simulink model "PI"  (R2020b)
settings: Solver=VariableStepAuto  StartTime=0.0  StopTime=300.0  RelTol=1e-3
values from neighbouring files (symbols this model uses):
  Kp = (0.9*T0)/(K0*(tau + 0.5*T)) - (0.5*Ki)/K0    (= 0.670050069403)    [Parametri_PI.m]    (also in Parametri_PID.m = 0.886775962404)
  T = 0.01    [Parametri_PI.m]    (also in Parametri_PID.m)
  Ti = (Kp*T)/Ki    (= 2.4575)    [Parametri_PI.m]    (also in Parametri_PID.m = 1.46356729475)
libraries: simulink x1
settings Model: Creator=user  LastModifiedBy=user

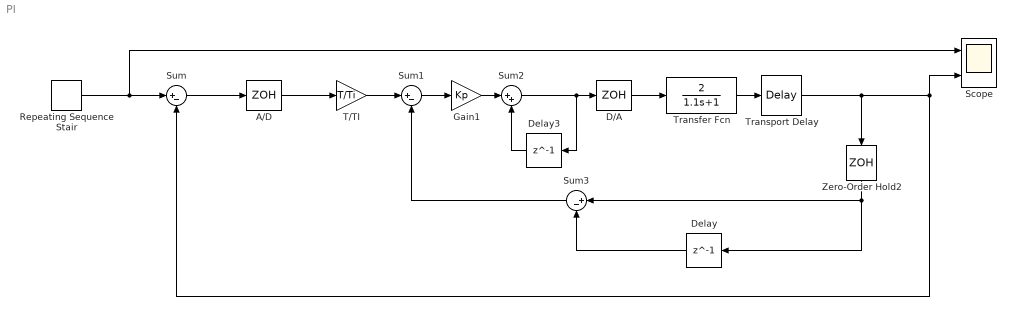
== system PI ==
  A/D : ZeroOrderHold  SampleTime=0.01
  D/A : ZeroOrderHold  SampleTime=0.01
  Delay : Delay  DelayLength=1
  Delay3 : Delay  DelayLength=1
  Gain1 : Gain  Gain=Kp
  Repeating Sequence Stair : simulink/Sources/Repeating Sequence Stair  OutValues=[3 1 -5 2 1].'  tsamp=50  OutMin=[]  OutMax=[]  OutDataTypeStr=double  OutputDataTypeScalingMode=double  OutDataType=fixdt(0,8)  ConRadixGroup=Best Precision: Vector-wise  OutScaling=2^-12
  Scope : Scope  NumInputPorts=2
  Sum : Sum  Inputs=|+-
  Sum1 : Sum  Inputs=|+-
  Sum2 : Sum  Inputs=|++
  Sum3 : Sum  Inputs=|+-
  T/TI : Gain  Gain=T/Ti
  Transfer Fcn : TransferFcn  Numerator=[2]  Denominator=[1.1 1]
  Transport Delay : TransportDelay  DelayTime=0.773
  Zero-Order Hold2 : ZeroOrderHold  SampleTime=0.01
  wires:
  Sum1/1 -> Gain1/1
  A/D/1 -> T/TI/1
  Delay/1 -> Sum3/2
  Transfer Fcn/1 -> Transport Delay/1
  Transport Delay/1 -> Sum/2, Scope/2, Zero-Order Hold2/1
  D/A/1 -> Transfer Fcn/1
  T/TI/1 -> Sum1/1
  Repeating Sequence Stair/1 -> Scope/1, Sum/1
  Gain1/1 -> Sum2/1
  Sum3/1 -> Sum1/2
  Zero-Order Hold2/1 -> Delay/1, Sum3/1
  Sum/1 -> A/D/1
  Delay3/1 -> Sum2/2
  Sum2/1 -> Delay3/1, D/A/1
